simulink model "MyInverseKinematics"  (R2021a)
settings: Solver=VariableStepAuto  StartTime=0.0  StopTime=10.0  RelTol=1e-3
settings Model: Creator=Al ien  LastModifiedBy=Al ien

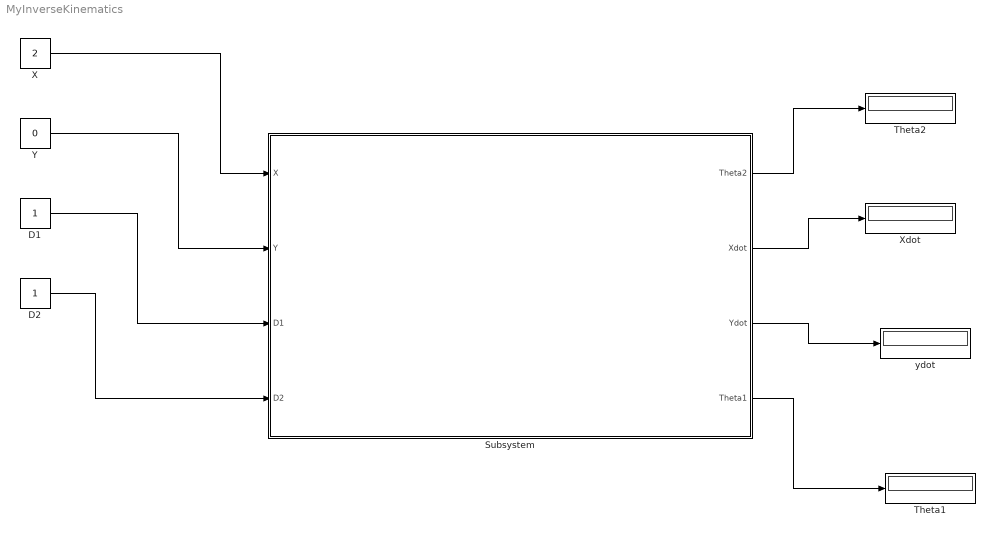
== system MyInverseKinematics ==
  D1 : Constant
  D2 : Constant
  Subsystem : Subsystem
  Theta1 : Display
  Theta2 : Display
  X : Constant  Value=2
  Xdot : Display
  Y : Constant  Value=0
  ydot : Display
  wires:
  X/1 -> Subsystem/1(X)
  Y/1 -> Subsystem/2(Y)
  D1/1 -> Subsystem/3(D1)
  D2/1 -> Subsystem/4(D2)
  Subsystem/1(Theta2) -> Theta2/1
  Subsystem/2(Xdot) -> Xdot/1
  Subsystem/3(Ydot) -> ydot/1
  Subsystem/4(Theta1) -> Theta1/1

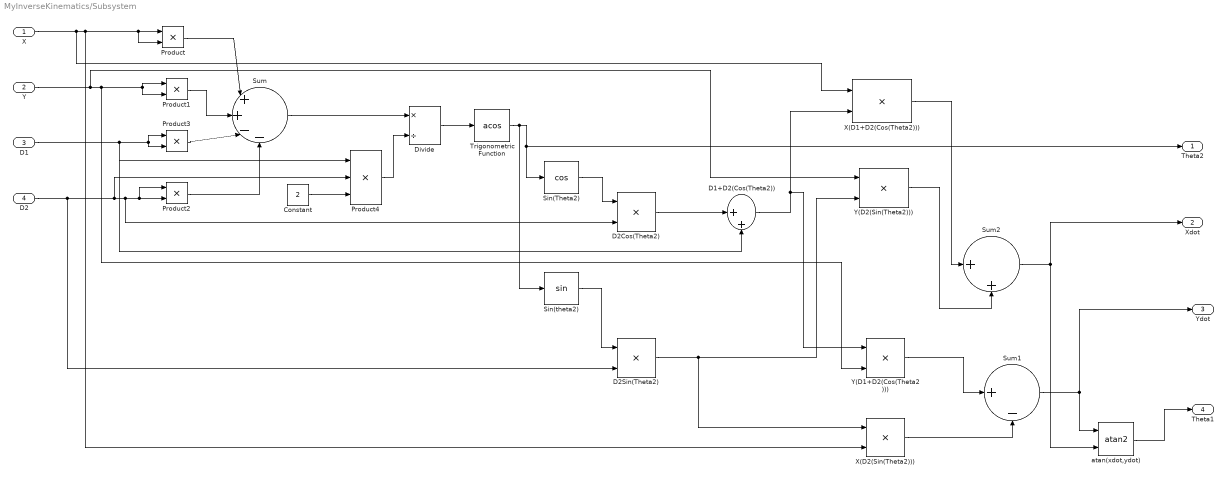
== system MyInverseKinematics/Subsystem ==
  X : Inport
  Y : Inport  Port=2
  D1 : Inport  Port=3
  D2 : Inport  Port=4
  Constant : Constant  Value=2
  D1+D2(Cos(Theta2)) : Sum  Inputs=|++
  D2Cos(Theta2) : Product
  D2Sin(Theta2) : Product
  Divide : Product  Inputs=*/
  Product{,1..3} (4 alike) : Product
  Product4 : Product  Inputs=3
  Sin(Theta2) : Trigonometry  Operator=cos
  Sin(theta2) : Trigonometry
  Sum : Sum  Inputs=|++--
  Sum1 : Sum  Inputs=|+-
  Sum2 : Sum  Inputs=|++
  Trigonometric Function : Trigonometry  Operator=acos
  X(D1+D2(Cos(Theta2))) : Product
  X(D2(Sin(Theta2))) : Product
  Y(D1+D2(Cos(Theta2))) : Product
  Y(D2(Sin(Theta2))) : Product
  atan(xdot,ydot) : Trigonometry  Operator=atan2
  Theta2 : Outport
  Xdot : Outport  Port=2
  Ydot : Outport  Port=3
  Theta1 : Outport  Port=4
  wires:
  D2Sin(Theta2)/1 -> X(D2(Sin(Theta2)))/1, Y(D2(Sin(Theta2)))/2
  Product1/1 -> Sum/2
  Sum/1 -> Divide/1
  Divide/1 -> Trigonometric Function/1
  Product/1 -> Sum/1
  Sin(theta2)/1 -> D2Sin(Theta2)/1
  D1+D2(Cos(Theta2))/1 -> Y(D1+D2(Cos(Theta2)))/1, X(D1+D2(Cos(Theta2)))/2
  Product4/1 -> Divide/2
  Product3/1 -> Sum/3
  Y(D2(Sin(Theta2)))/1 -> Sum2/2
  Y(D1+D2(Cos(Theta2)))/1 -> Sum1/1
  D1/1 -> D1+D2(Cos(Theta2))/2, Product3/2, Product3/1, Product4/1
  D2/1 -> D2Sin(Theta2)/2, Product4/2, D2Cos(Theta2)/2, Product2/1, Product2/2
  X/1 -> X(D1+D2(Cos(Theta2)))/1, X(D2(Sin(Theta2)))/2, Product/2, Product/1
  Sum1/1 -> Ydot/1, atan(xdot,ydot)/1
  Sin(Theta2)/1 -> D2Cos(Theta2)/1
  Sum2/1 -> Xdot/1, atan(xdot,ydot)/2
  X(D2(Sin(Theta2)))/1 -> Sum1/2
  Trigonometric Function/1 -> Sin(theta2)/1, Theta2/1, Sin(Theta2)/1
  Y/1 -> Y(D2(Sin(Theta2)))/1, Y(D1+D2(Cos(Theta2)))/2, Product1/1, Product1/2
  X(D1+D2(Cos(Theta2)))/1 -> Sum2/1
  D2Cos(Theta2)/1 -> D1+D2(Cos(Theta2))/1
  Product2/1 -> Sum/4
  Constant/1 -> Product4/3
  atan(xdot,ydot)/1 -> Theta1/1
